simulink model "Lidar_System_July11_NoPrintV1_Bayes_Sunny"  (Simulink 7.3)
settings: Solver=FixedStepDiscrete  StartTime=0.0  StopTime=inf  FixedStep=0.1  MaxStep=0.2  RelTol=1e-3
undefined symbols (not defined in the file): strel
libraries: dspmtrx3 x9, dspstat3 x4, simulink x3, vipstatistics x2, vipgeotforms x1, vipmorphops x1
(part 1 of 5)
settings Model: Creator=gclayton  LastModifiedBy=wildcat
settings DebuggingCC: InheritedTsInSrcMsg=none
settings RTWCC: SystemTargetFile=rlnx.tlc  GenCodeOnly=on  TemplateMakefile=rlnx_ubuntu.tmf  Description=Linux Real-Time Target  ProcessScript=rlnx_make_rtw_hook
settings RTWCC: CustomInclude=|
  | /usr/local/include/opencv/
  | /usr/local/include/
settings CodeAppCC: GenerateComments=off  SimulinkBlockComments=off
settings STFCustomTargetCC: ModelReferenceCompliant=off  MatFileLogging=on  SystemTargetFile=rlnx.tlc
settings GRTTargetCC: ModelReferenceCompliant=off  ParMdlRefBuildCompliant=off  CompOptLevelCompliant=off
settings CustomProperty: DataType=string  Value="-lm -ldl /usr/local/lib/libopencv_highgui.so.2.4 /usr/local/lib/libopencv_core.so.2.4 /usr/local/lib/libopencv_imgproc.so.2.4  -lc_urg -lc_urg_connection -lc_urg_system -lphidget21"
settings EnumStrPairs: String=PC

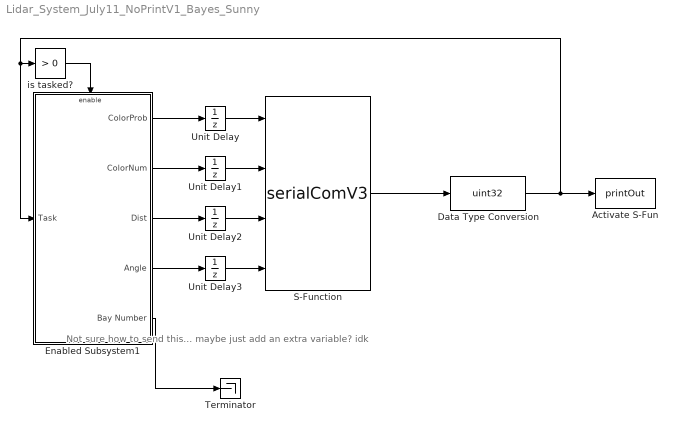
== system Lidar_System_July11_NoPrintV1_Bayes_Sunny ==
  note: Not sure how to
      | send this...
      | maybe just add an
      | extra variable? idk
  Activate S-Fun : S-Function  FunctionName=printOut  EnableBusSupport=off
  Data Type Conversion : DataTypeConversion  OutDataTypeMode=uint32  OutDataType=fixdt(1, 16)  OutScaling=2^0  OutDataTypeStr=uint32
  Enabled Subsystem1 : Subsystem  TreatAsAtomicUnit=on
  S-Function : S-Function  FunctionName=serialComV3  EnableBusSupport=off
  Terminator : Terminator
  Unit Delay : UnitDelay  SampleTime=-1
  Unit Delay1 : UnitDelay  X0=int32(0)  SampleTime=-1
  Unit Delay2 : UnitDelay  X0=int32(0)  SampleTime=-1
  Unit Delay3 : UnitDelay  X0=int32(0)  SampleTime=-1
  is tasked? : simulink/Logic and Bit Operations/Compare To Constant  SystemSampleTime=-1  relop=>  const=0  LogicOutDataTypeMode=uint8  ZeroCross=off
  wires:
  S-Function/1 -> Data Type Conversion/1
  Enabled Subsystem1/1(ColorProb) -> Unit Delay/1
  Enabled Subsystem1/2(ColorNum) -> Unit Delay1/1
  Enabled Subsystem1/3(Dist) -> Unit Delay2/1
  Enabled Subsystem1/4(Angle) -> Unit Delay3/1
  Unit Delay/1 -> S-Function/1
  Unit Delay1/1 -> S-Function/2
  Unit Delay2/1 -> S-Function/3
  Unit Delay3/1 -> S-Function/4
  Data Type Conversion/1 -> Activate S-Fun/1, Enabled Subsystem1/1(Task), is tasked?/1
  is tasked?/1 -> Enabled Subsystem1/Enable
  Enabled Subsystem1/5(Bay Number) -> Terminator/1

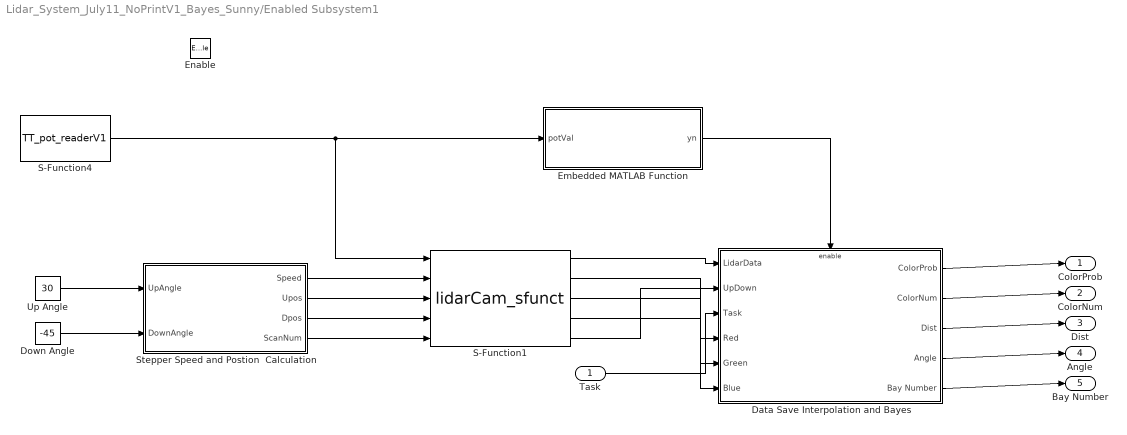
== system Lidar_System_July11_NoPrintV1_Bayes_Sunny/Enabled Subsystem1 ==
  Task : Inport  OutDataType=fixdt(1, 16)  OutScaling=2^0
  Enable : EnablePort
  Data Save Interpolation and Bayes : Subsystem  TreatAsAtomicUnit=on
  Down Angle : Constant  Value=-45  OutDataType=fixdt(1, 16)  OutScaling=2^0
  Embedded MATLAB Function : Stateflow chart
  S-Function1 : S-Function  FunctionName=lidarCam_sfunct  EnableBusSupport=off
  S-Function4 : S-Function  FunctionName=TT_pot_readerV1  EnableBusSupport=off
  Stepper Speed and Postion  Calculation : Stateflow chart
  Up Angle : Constant  Value=30  OutDataType=fixdt(1, 16)  OutScaling=2^0
  ColorProb : Outport  OutDataType=fixdt(1, 16)  OutScaling=2^0
  ColorNum : Outport  Port=2  OutDataType=fixdt(1, 16)  OutScaling=2^0
  Dist : Outport  Port=3  OutDataType=fixdt(1, 16)  OutScaling=2^0
  Angle : Outport  Port=4  OutDataType=fixdt(1, 16)  OutScaling=2^0
  Bay Number : Outport  Port=5  OutDataType=fixdt(1, 16)  OutScaling=2^0
  wires:
  S-Function4/1 -> S-Function1/1, Embedded MATLAB Function/1(potVal)
  Stepper Speed and Postion  Calculation/1(Speed) -> S-Function1/2
  Stepper Speed and Postion  Calculation/2(Upos) -> S-Function1/3
  Stepper Speed and Postion  Calculation/3(Dpos) -> S-Function1/4
  Stepper Speed and Postion  Calculation/4(ScanNum) -> S-Function1/5
  Embedded MATLAB Function/1(yn) -> Data Save Interpolation and Bayes/Enable
  S-Function1/1 -> Data Save Interpolation and Bayes/1(LidarData)
  Data Save Interpolation and Bayes/1(ColorProb) -> ColorProb/1
  Data Save Interpolation and Bayes/2(ColorNum) -> ColorNum/1
  Data Save Interpolation and Bayes/3(Dist) -> Dist/1
  Data Save Interpolation and Bayes/4(Angle) -> Angle/1
  Down Angle/1 -> Stepper Speed and Postion  Calculation/2(DownAngle)
  Up Angle/1 -> Stepper Speed and Postion  Calculation/1(UpAngle)
  Task/1 -> Data Save Interpolation and Bayes/3(Task)
  Data Save Interpolation and Bayes/5(Bay Number) -> Bay Number/1
  S-Function1/5 -> Data Save Interpolation and Bayes/2(UpDown)
  S-Function1/2 -> Data Save Interpolation and Bayes/4(Red)
  S-Function1/3 -> Data Save Interpolation and Bayes/5(Green)
  S-Function1/4 -> Data Save Interpolation and Bayes/6(Blue)

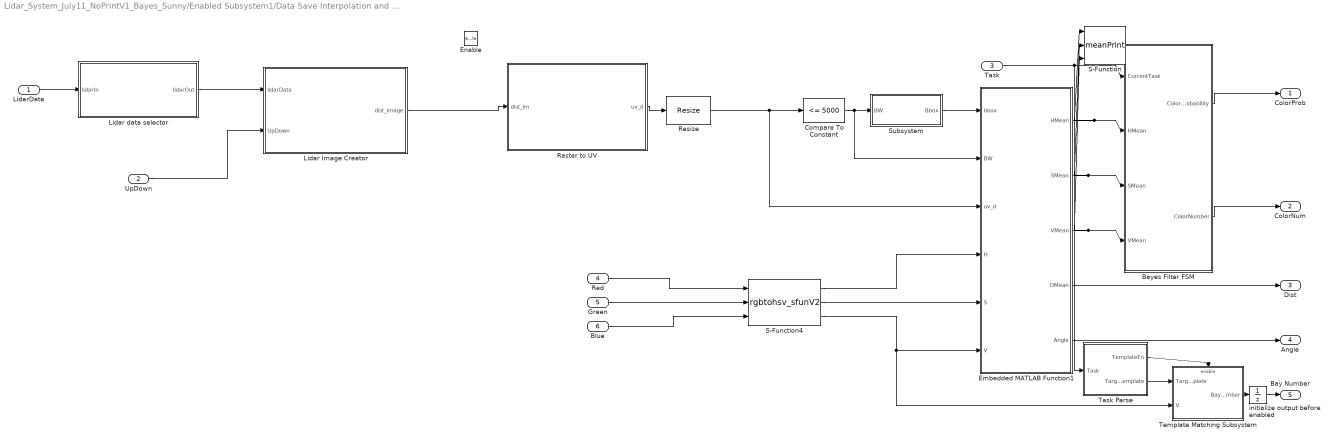
== system Lidar_System_July11_NoPrintV1_Bayes_Sunny/Enabled Subsystem1/Data Save Interpolation and Bayes ==
  LidarData : Inport  OutDataType=fixdt(1, 16)  OutScaling=2^0
  UpDown : Inport  Port=2  OutDataType=fixdt(1, 16)  OutScaling=2^0
  Task : Inport  Port=3  OutDataType=fixdt(1, 16)  OutScaling=2^0
  Red : Inport  Port=4  OutDataType=fixdt(1, 16)  OutScaling=2^0
  Green : Inport  Port=5  OutDataType=fixdt(1, 16)  OutScaling=2^0
  Blue : Inport  Port=6  OutDataType=fixdt(1, 16)  OutScaling=2^0
  Enable : EnablePort
  Bayes Filter FSM : Subsystem
  Compare To Constant : simulink/Logic and Bit Operations/Compare To Constant  SystemSampleTime=-1  relop=<=  const=5000  LogicOutDataTypeMode=boolean  ZeroCross=off
  Embedded MATLAB Function1 : Stateflow chart
  Lidar Image Creator : Stateflow chart
  Lidar data selector : Stateflow chart
  Raster to UV : Stateflow chart
  Resize : vipgeotforms/Resize  DialogController=vipDDGCreate  DialogControllerArgs=DataTag0  specify=Number of output rows and columns  rfactor=[200 150]  outCols=25  outRows=25  outRowsCols=[480 640]  interp_method=Bilinear  antialias=on  useROI=off  roiFlag=off  prodOutputMode=Binary point scaling  prodOutputWordLength=32  prodOutputFracLength=10  roundingMode=Nearest  overflowMode=on
  S-Function : S-Function  FunctionName=meanPrint  EnableBusSupport=off
  S-Function4 : S-Function  FunctionName=rgbtohsv_sfunV2  EnableBusSupport=off
  Subsystem : Subsystem
  Task Parse : Stateflow chart
  Template Matching Subsystem : Subsystem  TreatAsAtomicUnit=on
  initialize output before enabled : UnitDelay  SampleTime=-1
  ColorProb : Outport  OutDataType=fixdt(1, 16)  OutScaling=2^0
  ColorNum : Outport  Port=2  OutDataType=fixdt(1, 16)  OutScaling=2^0
  Dist : Outport  Port=3  OutDataType=fixdt(1, 16)  OutScaling=2^0
  Angle : Outport  Port=4  OutDataType=fixdt(1, 16)  OutScaling=2^0
  Bay Number : Outport  Port=5  OutDataType=fixdt(1, 16)  OutScaling=2^0
  wires:
  Lidar data selector/1(lidarOut) -> Lidar Image Creator/1(lidarData)
  UpDown/1 -> Lidar Image Creator/2(UpDown)
  Lidar Image Creator/1(dist_image) -> Raster to UV/1(dist_im)
  Compare To Constant/1 -> Subsystem/1(BW), Embedded MATLAB Function1/2(BW)
  Subsystem/1(Bbox) -> Embedded MATLAB Function1/1(bbox)
  Embedded MATLAB Function1/3(VMean) -> Bayes Filter FSM/4(VMean), S-Function/3
  Embedded MATLAB Function1/2(SMean) -> Bayes Filter FSM/3(SMean), S-Function/2
  Embedded MATLAB Function1/1(HMean) -> Bayes Filter FSM/2(HMean), S-Function/1
  Raster to UV/1(uv_d) -> Resize/1
  Bayes Filter FSM/1(ColorProbability) -> ColorProb/1
  Bayes Filter FSM/2(ColorNumber) -> ColorNum/1
  Embedded MATLAB Function1/5(Angle) -> Angle/1
  Embedded MATLAB Function1/4(DMean) -> Dist/1
  Red/1 -> S-Function4/1
  Green/1 -> S-Function4/2
  Blue/1 -> S-Function4/3
  S-Function4/1 -> Embedded MATLAB Function1/4(H)
  S-Function4/2 -> Embedded MATLAB Function1/5(S)
  S-Function4/3 -> Embedded MATLAB Function1/6(V), Template Matching Subsystem/2(V)
  LidarData/1 -> Lidar data selector/1(lidarIn)
  Resize/1 -> Compare To Constant/1, Embedded MATLAB Function1/3(uv_d)
  Task Parse/1(TemplateEn) -> Template Matching Subsystem/Enable
  Task Parse/2(TargetTemplate) -> Template Matching Subsystem/1(Target Template)
  Template Matching Subsystem/1(Bay Number) -> initialize output before enabled/1
  initialize output before enabled/1 -> Bay Number/1
  Task/1 -> Bayes Filter FSM/1(CurrentTask), Task Parse/1(Task)

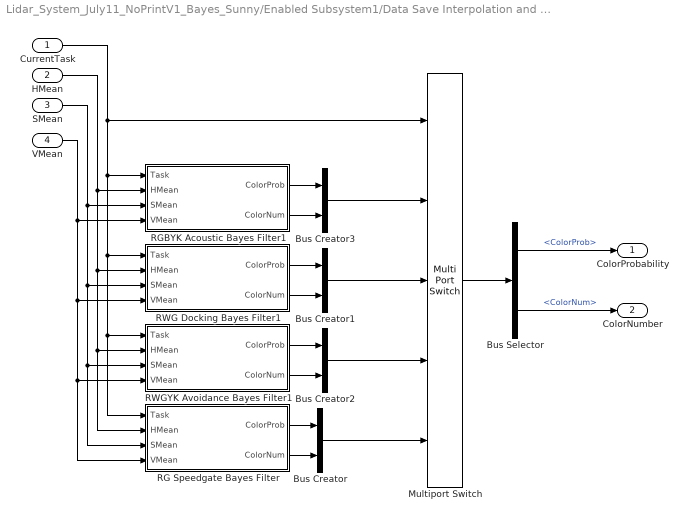
== system Lidar_System_July11_NoPrintV1_Bayes_Sunny/Enabled Subsystem1/Data Save Interpolation and Bayes/Bayes Filter FSM ==
  CurrentTask : Inport  OutDataType=fixdt(1, 16)  OutScaling=2^0
  HMean : Inport  Port=2  OutDataType=fixdt(1, 16)  OutScaling=2^0
  SMean : Inport  Port=3  OutDataType=fixdt(1, 16)  OutScaling=2^0
  VMean : Inport  Port=4  OutDataType=fixdt(1, 16)  OutScaling=2^0
  Bus Creator{,1..3} (4 alike) : BusCreator  Inputs=2
  Bus Selector : BusSelector  OutputSignals=ColorProb,ColorNum
  Multiport Switch : MultiPortSwitch  Inputs=4  OutDataType=fixdt(1, 16)  OutScaling=2^0
  RG Speedgate Bayes Filter : Stateflow chart
  RGBYK Acoustic Bayes Filter1 : Stateflow chart
  RWG Docking Bayes Filter1 : Stateflow chart
  RWGYK Avoidance Bayes Filter1 : Stateflow chart
  ColorProbability : Outport  OutDataType=fixdt(1, 16)  OutScaling=2^0
  ColorNumber : Outport  Port=2  OutDataType=fixdt(1, 16)  OutScaling=2^0
  wires:
  RWG Docking Bayes Filter1/1(ColorProb) -> Bus Creator1/1
  RWG Docking Bayes Filter1/2(ColorNum) -> Bus Creator1/2
  RWGYK Avoidance Bayes Filter1/1(ColorProb) -> Bus Creator2/1
  RWGYK Avoidance Bayes Filter1/2(ColorNum) -> Bus Creator2/2
  Bus Creator1/1 -> Multiport Switch/3
  Bus Creator2/1 -> Multiport Switch/4
  HMean/1 -> RWG Docking Bayes Filter1/2(HMean), RWGYK Avoidance Bayes Filter1/2(HMean), RG Speedgate Bayes Filter/2(HMean), RGBYK Acoustic Bayes Filter1/2(HMean)
  SMean/1 -> RWG Docking Bayes Filter1/3(SMean), RWGYK Avoidance Bayes Filter1/3(SMean), RG Speedgate Bayes Filter/3(SMean), RGBYK Acoustic Bayes Filter1/3(SMean)
  VMean/1 -> RWG Docking Bayes Filter1/4(VMean), RWGYK Avoidance Bayes Filter1/4(VMean), RG Speedgate Bayes Filter/4(VMean), RGBYK Acoustic Bayes Filter1/4(VMean)
  Multiport Switch/1 -> Bus Selector/1
  Bus Selector/1 -> ColorProbability/1  "<ColorProb>"
  Bus Selector/2 -> ColorNumber/1  "<ColorNum>"
  CurrentTask/1 -> RWG Docking Bayes Filter1/1(Task), RWGYK Avoidance Bayes Filter1/1(Task), RG Speedgate Bayes Filter/1(Task), RGBYK Acoustic Bayes Filter1/1(Task), Multiport Switch/1
  RG Speedgate Bayes Filter/1(ColorProb) -> Bus Creator/1
  RG Speedgate Bayes Filter/2(ColorNum) -> Bus Creator/2
  RGBYK Acoustic Bayes Filter1/1(ColorProb) -> Bus Creator3/1
  RGBYK Acoustic Bayes Filter1/2(ColorNum) -> Bus Creator3/2
  Bus Creator3/1 -> Multiport Switch/2
  Bus Creator/1 -> Multiport Switch/5

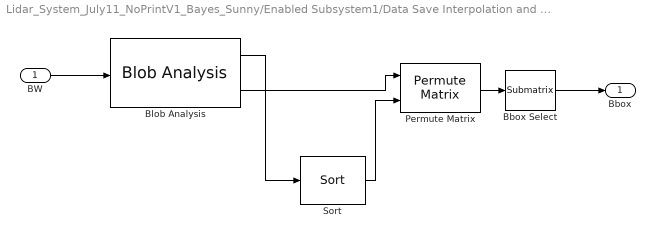
== system Lidar_System_July11_NoPrintV1_Bayes_Sunny/Enabled Subsystem1/Data Save Interpolation and Bayes/Subsystem ==
  BW : Inport  OutDataType=fixdt(1, 16)  OutScaling=2^0
  Bbox Select : dspmtrx3/Submatrix  RowSpan=All rows  RowStartMode=First  RowStartIndex=1  RowEndMode=Last  RowEndIndex=1  ColSpan=One column  ColStartMode=First  ColStartIndex=1  ColEndMode=Last  ColEndIndex=1
  Blob Analysis : vipstatistics/Blob Analysis  DialogController=vipDDGCreate  DialogControllerArgs=DataTag1  area=on  centroid=off  bBox=on  majorAxis=off  minorAxis=off  angle=off  eccentricity=off  equivDiameterSq=off  extent=off  perimeter=off  maxBlobs=20  warnIfNumBlobsExceeded=on  isCount=off  useMinArea=on  minArea=20  useMaxArea=off  maxArea=intmax('uint32')  excludeBorderBlob=off  outDT=double  isOutVarDim=off  isFill=on  fillValues=-1  conn=8  isLabel=off  outputMode=Binary point scaling  outputWordLength=32  outputFracLength=16  firstCoeffMode=Binary point scaling  firstCoeffWordLength=16  firstCoeffFracLength=14  secondCoeffMode=Binary point scaling  secondCoeffWordLength=32  secondCoeffFracLength=16  accumMode=Binary point scaling  accumWordLength=32  accumFracLength=0  prodOutputMode=Binary point scaling  prodOutputWordLength=32  prodOutputFracLength=16  roundingMode=Floor  overflowMode=off
  Permute Matrix : dspmtrx3/Permute Matrix  mode=Columns  ZeroOneIdxMode=One-based  errmode=Clip index  checkDims=off
  Sort : dspstat3/Sort  DialogController=dspDDGCreate  DialogControllerArgs=DataTag2  otype=Index  dir=Descending  sortAlg=Quick sort  roundingMode=Floor  overflowMode=off
  Bbox : Outport  OutDataType=fixdt(1, 16)  OutScaling=2^0
  wires:
  BW/1 -> Blob Analysis/1
  Blob Analysis/1 -> Sort/1
  Sort/1 -> Permute Matrix/2
  Blob Analysis/2 -> Permute Matrix/1
  Permute Matrix/1 -> Bbox Select/1
  Bbox Select/1 -> Bbox/1

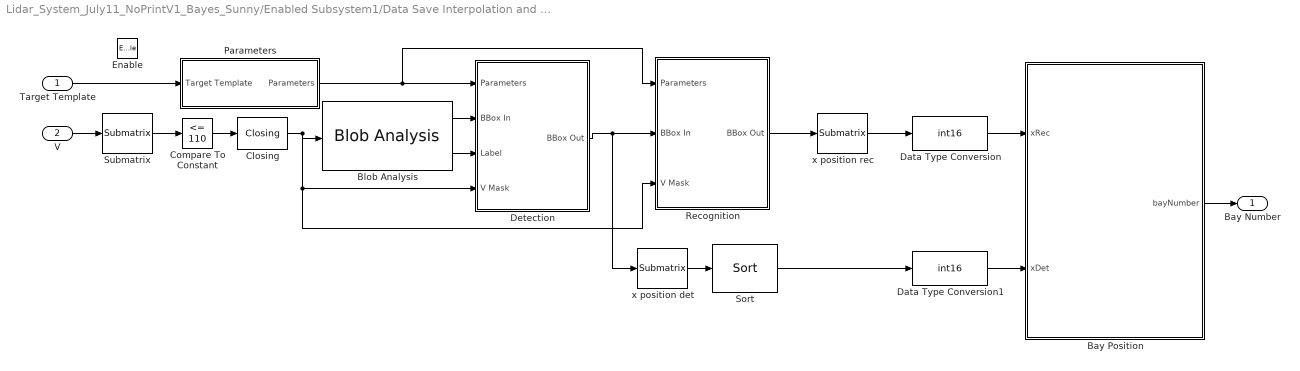
== system Lidar_System_July11_NoPrintV1_Bayes_Sunny/Enabled Subsystem1/Data Save Interpolation and Bayes/Template Matching Subsystem ==
  Target Template : Inport  OutDataType=fixdt(1, 16)  OutScaling=2^0
  V : Inport  Port=2  OutDataType=fixdt(1, 16)  OutScaling=2^0
  Enable : EnablePort
  Bay Position : Stateflow chart
  Blob Analysis : vipstatistics/Blob Analysis  DialogController=vipDDGCreate  DialogControllerArgs=DataTag3  area=off  centroid=off  bBox=on  majorAxis=off  minorAxis=off  angle=off  eccentricity=off  equivDiameterSq=off  extent=off  perimeter=off  maxBlobs=10  warnIfNumBlobsExceeded=on  isCount=off  useMinArea=on  minArea=700  useMaxArea=off  maxArea=intmax('uint32')  excludeBorderBlob=on  outDT=double  isOutVarDim=off  isFill=on  fillValues=-1  conn=8  isLabel=on  outputMode=Binary point scaling  outputWordLength=32  outputFracLength=16  firstCoeffMode=Binary point scaling  firstCoeffWordLength=16  firstCoeffFracLength=14  secondCoeffMode=Binary point scaling  secondCoeffWordLength=32  secondCoeffFracLength=16  accumMode=Binary point scaling  accumWordLength=32  accumFracLength=0  prodOutputMode=Binary point scaling  prodOutputWordLength=32  prodOutputFracLength=16  roundingMode=Floor  overflowMode=off
  Closing : vipmorphops/Closing  nhoodsrc=Specify via dialog  strel=strel('disk',1,4)
  Compare To Constant : simulink/Logic and Bit Operations/Compare To Constant  SystemSampleTime=-1  relop=<=  const=110  LogicOutDataTypeMode=boolean  ZeroCross=off
  Data Type Conversion : DataTypeConversion  OutDataTypeMode=int16  OutDataType=fixdt(1, 16)  OutScaling=2^0  OutDataTypeStr=int16
  Data Type Conversion1 : DataTypeConversion  OutDataTypeMode=int16  OutDataType=fixdt(1, 16)  OutScaling=2^0  OutDataTypeStr=int16
  Detection : Subsystem
  Parameters : Subsystem
  Recognition : Subsystem
  Sort : dspstat3/Sort  DialogController=dspDDGCreate  DialogControllerArgs=DataTag6  otype=Value  dir=Ascending  sortAlg=Quick sort  roundingMode=Floor  overflowMode=off
  Submatrix : dspmtrx3/Submatrix  RowSpan=Range of rows  RowStartMode=First  RowStartIndex=1  RowEndMode=Index  RowEndIndex=240  ColSpan=Range of columns  ColStartMode=First  ColStartIndex=1  ColEndMode=Last  ColEndIndex=1
  x position det : dspmtrx3/Submatrix  RowSpan=One row  RowStartMode=Index  RowStartIndex=2  RowEndMode=Last  RowEndIndex=1  ColSpan=Range of columns  ColStartMode=First  ColStartIndex=1  ColEndMode=Last  ColEndIndex=1
  x position rec : dspmtrx3/Submatrix  RowSpan=One row  RowStartMode=Index  RowStartIndex=2  RowEndMode=Last  RowEndIndex=1  ColSpan=Range of columns  ColStartMode=First  ColStartIndex=1  ColEndMode=Last  ColEndIndex=1
  Bay Number : Outport  OutDataType=fixdt(1, 16)  OutScaling=2^0
  wires:
  V/1 -> Submatrix/1
  Submatrix/1 -> Compare To Constant/1
  Compare To Constant/1 -> Closing/1
  Closing/1 -> Blob Analysis/1, Detection/4(V Mask), Recognition/3(V Mask)
  Blob Analysis/1 -> Detection/2(BBox In)
  Blob Analysis/2 -> Detection/3(Label)
  Target Template/1 -> Parameters/1(Target Template)
  Parameters/1(Parameters) -> Detection/1(Parameters), Recognition/1(Parameters)
  Detection/1(BBox Out) -> Recognition/2(BBox In), x position det/1
  x position det/1 -> Sort/1
  Recognition/1(BBox Out) -> x position rec/1
  x position rec/1 -> Data Type Conversion/1
  Sort/1 -> Data Type Conversion1/1
  Data Type Conversion/1 -> Bay Position/1(xRec)
  Data Type Conversion1/1 -> Bay Position/2(xDet)
  Bay Position/1(bayNumber) -> Bay Number/1

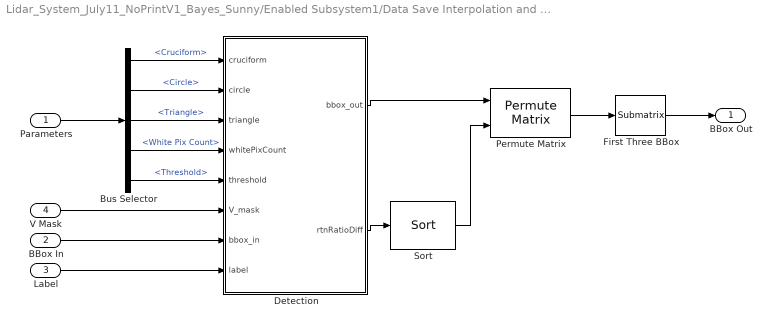
== system Lidar_System_July11_NoPrintV1_Bayes_Sunny/Enabled Subsystem1/Data Save Interpolation and Bayes/Template Matching Subsystem/Detection ==
  Parameters : Inport  OutDataType=fixdt(1, 16)  OutScaling=2^0
  BBox In : Inport  Port=2  OutDataType=fixdt(1, 16)  OutScaling=2^0
  Label : Inport  Port=3  OutDataType=fixdt(1, 16)  OutScaling=2^0
  V Mask : Inport  Port=4  OutDataType=fixdt(1, 16)  OutScaling=2^0
  Bus Selector : BusSelector  OutputSignals=Templates.Cruciform,Templates.Circle,Templates.Triangle,White Pix Count,Threshold
  Detection : Stateflow chart
  First Three BBox : dspmtrx3/Submatrix  RowSpan=All rows  RowStartMode=First  RowStartIndex=1  RowEndMode=Last  RowEndIndex=1  ColSpan=Range of columns  ColStartMode=First  ColStartIndex=1  ColEndMode=Index  ColEndIndex=3
  Permute Matrix : dspmtrx3/Permute Matrix  mode=Columns  ZeroOneIdxMode=One-based  errmode=Clip index  checkDims=off
  Sort : dspstat3/Sort  DialogController=dspDDGCreate  DialogControllerArgs=DataTag4  otype=Index  dir=Ascending  sortAlg=Quick sort  roundingMode=Floor  overflowMode=off
  BBox Out : Outport  OutDataType=fixdt(1, 16)  OutScaling=2^0
  wires:
  Parameters/1 -> Bus Selector/1
  Bus Selector/1 -> Detection/1(cruciform)  "<Cruciform>"
  Bus Selector/2 -> Detection/2(circle)  "<Circle>"
  Bus Selector/3 -> Detection/3(triangle)  "<Triangle>"
  Bus Selector/4 -> Detection/4(whitePixCount)  "<White Pix Count>"
  Bus Selector/5 -> Detection/5(threshold)  "<Threshold>"
  Label/1 -> Detection/8(label)
  BBox In/1 -> Detection/7(bbox_in)
  V Mask/1 -> Detection/6(V_mask)
  Detection/2(rtnRatioDiff) -> Sort/1
  Detection/1(bbox_out) -> Permute Matrix/1
  Sort/1 -> Permute Matrix/2
  Permute Matrix/1 -> First Three BBox/1
  First Three BBox/1 -> BBox Out/1

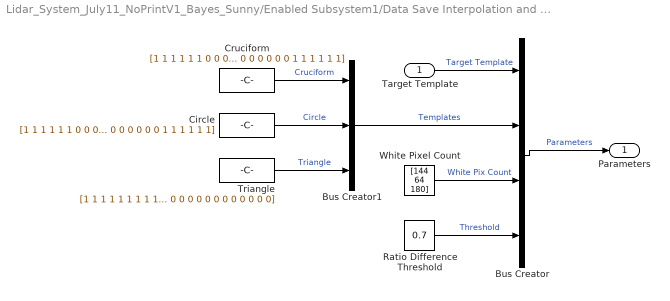
== system Lidar_System_July11_NoPrintV1_Bayes_Sunny/Enabled Subsystem1/Data Save Interpolation and Bayes/Template Matching Subsystem/Parameters ==
  Target Template : Inport  OutDataType=fixdt(1, 16)  OutScaling=2^0
  Bus Creator : BusCreator
  Bus Creator1 : BusCreator  Inputs=3
  Circle : Constant  Value=|  OutDataType=fixdt(1, 16)  OutScaling=2^0
      | [1	1	1	1	1	1	0	0	0	0	0	0	0	1	1	1	1	1	1
      | 1	1	1	1	0	0	0	0	0	0	0	0	0	0	0	1	1	1	1
      | 1	1	0	0	0	0	0	0	0	0	0	0	0	0	0	0	0	1	1
      | 1	1	0	0	0	0	0	0	0	0	0	0	0	0	0	0	0	1	1
      | 1	0	0	0	0	0	0	0	0	0	0	0	0	0	0	0	0	0	1
      | 1	0	0	0	0	0	0	0	0	0	0	0	0	0	0	0	0	0	1
      | 0	0	0	0	0	0	0	0	0	0	0	0	0	0	0	0	0	0	0
      | 0	0	0	0	0	0	0	0	0	0	0	0	0	0	0	0	0	0	0
      | 0	0	0	0	0	0	0	0	0	0	0	0	0	0	0	0	0	0	0
      | 0	0	0	0	0	0	0	0	0	0	0	0	0	0	0	0	0	0	0
      | 0	0	0	0	0	0	0	0	0	0	0	0	0	0	0	0	0	0	0
      | 0	0	0	0	0	0	0	0	0	0	0	0	0	0	0	0	0	0	0
      | 0	0	0	0	0	0	0	0	0	0	0	0	0	0	0	0	0	0	0
      | 1	0	0	0	0	0	0	0	0	0	0	0	0	0	0	0	0	0	1
      | 1	0	0	0	0	0	0	0	0	0	0	0	0	0	0	0	0	0	1
      | 1	1	0	0	0	0	0	0	0	0	0	0	0	0	0	0	0	1	1
      | 1	1	0	0	0	0	0	0	0	0	0	0	0	0	0	0	0	1	1
      | 1	1	1	1	0	0	0	0	0	0	0	0	0	0	0	1	1	1	1
      | 1	1	1	1	1	1	0	0	0	0	0	0	0	1	1	1	1	1	1]
  Cruciform : Constant  Value=|  OutDataType=fixdt(1, 16)  OutScaling=2^0
      | [1	1	1	1	1	1	0	0	0	0	0	0	0	1	1	1	1	1	1
      | 1	1	1	1	1	1	0	0	0	0	0	0	0	1	1	1	1	1	1
      | 1	1	1	1	1	1	0	0	0	0	0	0	0	1	1	1	1	1	1
      | 1	1	1	1	1	1	0	0	0	0	0	0	0	1	1	1	1	1	1
      | 1	1	1	1	1	1	0	0	0	0	0	0	0	1	1	1	1	1	1
      | 1	1	1	1	1	1	0	0	0	0	0	0	0	1	1	1	1	1	1
      | 0	0	0	0	0	0	0	0	0	0	0	0	0	0	0	0	0	0	0
      | 0	0	0	0	0	0	0	0	0	0	0	0	0	0	0	0	0	0	0
      | 0	0	0	0	0	0	0	0	0	0	0	0	0	0	0	0	0	0	0
      | 0	0	0	0	0	0	0	0	0	0	0	0	0	0	0	0	0	0	0
      | 0	0	0	0	0	0	0	0	0	0	0	0	0	0	0	0	0	0	0
      | 0	0	0	0	0	0	0	0	0	0	0	0	0	0	0	0	0	0	0
      | 0	0	0	0	0	0	0	0	0	0	0	0	0	0	0	0	0	0	0
      | 1	1	1	1	1	1	0	0	0	0	0	0	0	1	1	1	1	1	1
      | 1	1	1	1	1	1	0	0	0	0	0	0	0	1	1	1	1	1	1
      | 1	1	1	1	1	1	0	0	0	0	0	0	0	1	1	1	1	1	1
      | 1	1	1	1	1	1	0	0	0	0	0	0	0	1	1	1	1	1	1
      | 1	1	1	1	1	1	0	0	0	0	0	0	0	1	1	1	1	1	1
      | 1	1	1	1	1	1	0	0	0	0	0	0	0	1	1	1	1	1	1]
  Ratio Difference Threshold : Constant  Value=0.7  OutDataType=fixdt(1, 16)  OutScaling=2^0
  Triangle : Constant  Value=|  OutDataType=fixdt(1, 16)  OutScaling=2^0
      | [1	1	1	1	1	1	1	1	1	0	1	1	1	1	1	1	1	1	1
      | 1	1	1	1	1	1	1	1	1	0	1	1	1	1	1	1	1	1	1
      | 1	1	1	1	1	1	1	1	0	0	0	1	1	1	1	1	1	1	1
      | 1	1	1	1	1	1	1	1	0	0	0	1	1	1	1	1	1	1	1
      | 1	1	1	1	1	1	1	0	0	0	0	0	1	1	1	1	1	1	1
      | 1	1	1	1	1	1	1	0	0	0	0	0	1	1	1	1	1	1	1
      | 1	1	1	1	1	1	0	0	0	0	0	0	0	1	1	1	1	1	1
      | 1	1	1	1	1	1	0	0	0	0	0	0	0	1	1	1	1	1	1
      | 1	1	1	1	1	0	0	0	0	0	0	0	0	0	1	1	1	1	1
      | 1	1	1	1	1	0	0	0	0	0	0	0	0	0	1	1	1	1	1
      | 1	1	1	1	0	0	0	0	0	0	0	0	0	0	0	1	1	1	1
      | 1	1	1	1	0	0	0	0	0	0	0	0	0	0	0	1	1	1	1
      | 1	1	1	0	0	0	0	0	0	0	0	0	0	0	0	0	1	1	1
      | 1	1	1	0	0	0	0	0	0	0	0	0	0	0	0	0	1	1	1
      | 1	1	0	0	0	0	0	0	0	0	0	0	0	0	0	0	0	1	1
      | 1	1	0	0	0	0	0	0	0	0	0	0	0	0	0	0	0	1	1
      | 1	0	0	0	0	0	0	0	0	0	0	0	0	0	0	0	0	0	1
      | 1	0	0	0	0	0	0	0	0	0	0	0	0	0	0	0	0	0	1
      | 0	0	0	0	0	0	0	0	0	0	0	0	0	0	0	0	0	0	0]
  White Pixel Count : Constant  Value=[144 64 180]  OutDataType=fixdt(1, 16)  OutScaling=2^0
  Parameters : Outport  OutDataType=fixdt(1, 16)  OutScaling=2^0
  wires:
  Target Template/1 -> Bus Creator/1  "Target Template"
  White Pixel Count/1 -> Bus Creator/3  "White Pix Count"
  Ratio Difference Threshold/1 -> Bus Creator/4  "Threshold"
  Bus Creator1/1 -> Bus Creator/2  "Templates"
  Cruciform/1 -> Bus Creator1/1  "Cruciform"
  Circle/1 -> Bus Creator1/2  "Circle"
  Triangle/1 -> Bus Creator1/3  "Triangle"
  Bus Creator/1 -> Parameters/1  "Parameters"

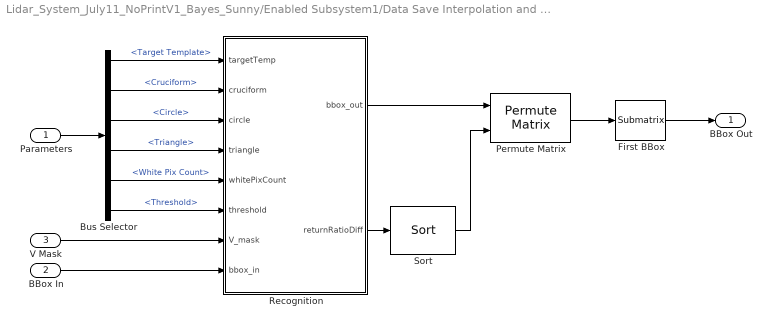
== system Lidar_System_July11_NoPrintV1_Bayes_Sunny/Enabled Subsystem1/Data Save Interpolation and Bayes/Template Matching Subsystem/Recognition ==
  Parameters : Inport  OutDataType=fixdt(1, 16)  OutScaling=2^0
  BBox In : Inport  Port=2  OutDataType=fixdt(1, 16)  OutScaling=2^0
  V Mask : Inport  Port=3  OutDataType=fixdt(1, 16)  OutScaling=2^0
  Bus Selector : BusSelector  OutputSignals=Target Template,Templates.Cruciform,Templates.Circle,Templates.Triangle,White Pix Count,Threshold
  First BBox : dspmtrx3/Submatrix  RowSpan=All rows  RowStartMode=First  RowStartIndex=1  RowEndMode=Last  RowEndIndex=1  ColSpan=One column  ColStartMode=First  ColStartIndex=1  ColEndMode=Index  ColEndIndex=3
  Permute Matrix : dspmtrx3/Permute Matrix  mode=Columns  ZeroOneIdxMode=One-based  errmode=Clip index  checkDims=off
  Recognition : Stateflow chart
  Sort : dspstat3/Sort  DialogController=dspDDGCreate  DialogControllerArgs=DataTag5  otype=Index  dir=Ascending  sortAlg=Quick sort  roundingMode=Floor  overflowMode=off
  BBox Out : Outport  OutDataType=fixdt(1, 16)  OutScaling=2^0
  wires:
  Parameters/1 -> Bus Selector/1
  Bus Selector/2 -> Recognition/2(cruciform)  "<Cruciform>"
  Bus Selector/3 -> Recognition/3(circle)  "<Circle>"
  Bus Selector/4 -> Recognition/4(triangle)  "<Triangle>"
  Bus Selector/5 -> Recognition/5(whitePixCount)  "<White Pix Count>"
  Bus Selector/6 -> Recognition/6(threshold)  "<Threshold>"
  BBox In/1 -> Recognition/8(bbox_in)
  V Mask/1 -> Recognition/7(V_mask)
  Recognition/2(returnRatioDiff) -> Sort/1
  Recognition/1(bbox_out) -> Permute Matrix/1
  Sort/1 -> Permute Matrix/2
  Permute Matrix/1 -> First BBox/1
  First BBox/1 -> BBox Out/1
  Bus Selector/1 -> Recognition/1(targetTemp)  "<Target Template>"
